simulink model "Modelo_controlador_estados"  (R2021a)
settings: Solver=FixedStepAuto  StartTime=0.0  StopTime=3  FixedStep=0.001  RelTol=1e-3
libraries: simulink x1
settings Model: Creator=faust  LastModifiedBy=joaqu

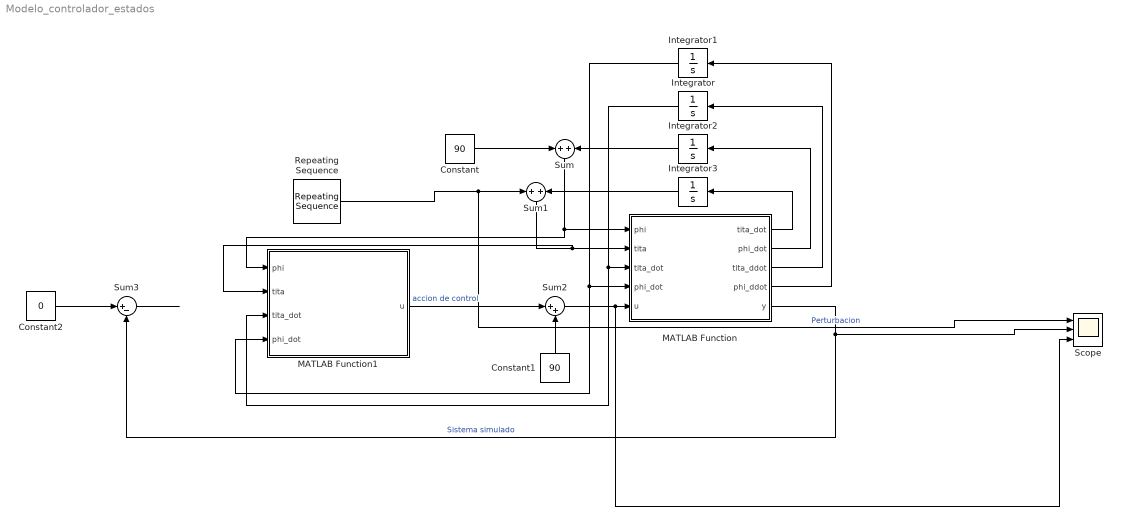
== system Modelo_controlador_estados ==
  Constant : Constant  Value=90
  Constant1 : Constant  Value=90
  Constant2 : Constant  Value=0
  Integrator{,1..3} (4 alike) : Integrator
  MATLAB Function : MATLAB Function  TreatAsAtomicUnit=on
  MATLAB Function1 : MATLAB Function  TreatAsAtomicUnit=on
  Repeating Sequence : simulink/Sources/Repeating Sequence  rep_seq_t=[0 0.08 0.24 0.25 0.36 5]  rep_seq_y=[0 0 30 0 0 0]
  Scope : Scope  NumInputPorts=3
  Sum : Sum  Inputs=+|+
  Sum1 : Sum  Inputs=+|+
  Sum2 : Sum  Inputs=|++
  Sum3 : Sum  Inputs=|+-
  wires:
  MATLAB Function/3(tita_ddot) -> Integrator/1
  Integrator/1 -> MATLAB Function1/3(tita_dot), MATLAB Function/3("tita_dot ")
  MATLAB Function/5(y) -> Sum3/2, Scope/2  "Sistema simulado"
  MATLAB Function/4(phi_ddot) -> Integrator1/1
  Integrator1/1 -> MATLAB Function1/4(phi_dot), MATLAB Function/4("phi_dot ")
  MATLAB Function/1(tita_dot) -> Integrator3/1
  MATLAB Function/2(phi_dot) -> Integrator2/1
  Sum1/1 -> MATLAB Function1/2(tita), MATLAB Function/2(tita)
  Integrator3/1 -> Sum1/2
  Constant/1 -> Sum/1
  Sum/1 -> MATLAB Function1/1(phi), MATLAB Function/1(phi)
  Integrator2/1 -> Sum/2
  Constant2/1 -> Sum3/1
  MATLAB Function1/1(u) -> Sum2/1  "accion de control"
  Constant1/1 -> Sum2/2
  Sum3/1 -> ?
  Repeating Sequence/1 -> Scope/1, Sum1/1  "Perturbacion"
  Sum2/1 -> Scope/3, MATLAB Function/5(u)

== matlab function Modelo_controlador_estados/MATLAB Function1 ==
  data: u output; phi input; tita input; tita_dot input; phi_dot input
function u = fcn(phi, tita, tita_dot,phi_dot)

K = [-0.9757, 0.0129, 0.7346, -0.0115];

phi_eq = 90;

u = K(1) * tita + K(2) * tita_dot + K(3) * (phi - phi_eq) + K(4) * phi_dot;

== matlab function Modelo_controlador_estados/MATLAB Function ==
  data: tita_dot output; phi_dot output; phi input; tita input; tita_dot input; phi_dot input; tita_ddot output; phi_ddot output; u input; y output
function [tita_dot,phi_dot,tita_ddot,phi_ddot,y] = fcn(phi, tita, tita_dot,phi_dot,u)

a = 0.7;
b = 2.613;
c = 65;
d = 292.2;
e = 30.67;
f = d;

phi_ddot = d * u - e * phi_dot - f * phi;
tita_ddot = - b * tita_dot - c * tita - a*f * phi - a * e * phi_dot + a * d *u;

y = tita;
